simulink model "EV_Model"  (R2023b)
settings: Solver=FixedStepAuto  StartTime=0.0  StopTime=100  FixedStep=0.01  RelTol=1e-3
values from neighbouring files (symbols this model uses):
  Area = 2.3    [Data.m]
  Cd = 0.28    [Data.m]
  f = 0.01    [Data.m]
  g = 9.8    [Data.m]
  GearEff = 0.97    [Data.m]
  GearRto = 9.7    [Data.m]
  Grad = 0    [Data.m]
  MotDrvCrv_1X_rpm = [1000 2000 3000 4000 5000 6000 7000 8000 9000 10000 12000 13000 14000 15000 16000]    [Data.m]
  MotDrvCrv_1Y_Tq = [390 390 390 389 311 259 222 195 173 156 142 130 120 111 104]    [Data.m]
  MotGenCrv_1X_rpm = MotDrvCrv_1X_rpm    [Data.m]
  MotGenCrv_1Y_Tq = -1*MotDrvCrv_1Y_Tq    [Data.m]
  RotCoeff = 0.05    [Data.m]
  vhemass = 1500    [Data.m]
  WhlRollRads = 0.327    [Data.m]
libraries: simulink x2
settings Model: Creator=bingtao.hu  LastModifiedBy=bingtao.hu

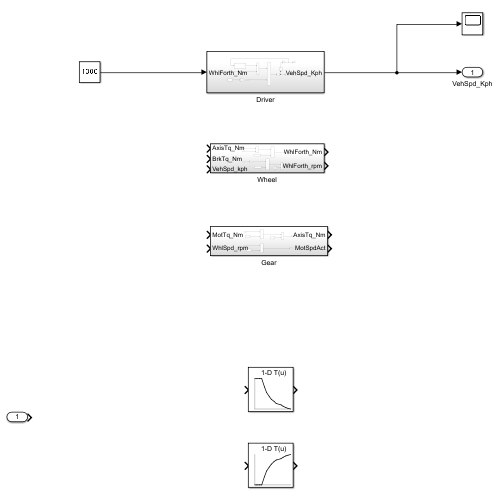
[thumbnail: Simulink's stored preview of the top-level diagram]
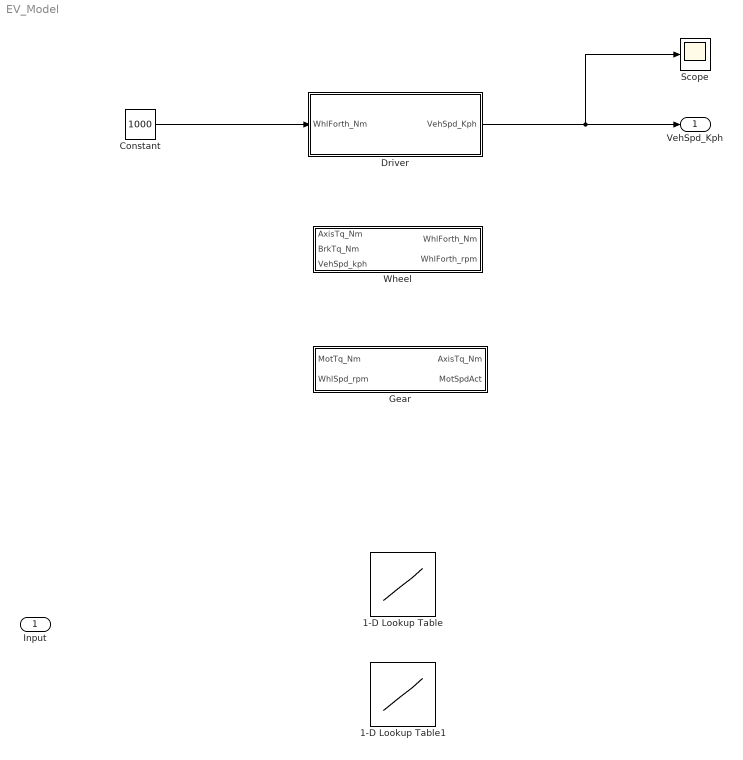
== system EV_Model ==
  Input : Inport
  1-D Lookup Table : Lookup_n-D  NumberOfTableDimensions=1  BreakpointsForDimension1=MotDrvCrv_1X_rpm  Table=MotDrvCrv_1Y_Tq  ExtrapMethod=Clip  UseLastTableValue=on  InternalRulePriority=Speed  RndMeth=Simplest
  1-D Lookup Table1 : Lookup_n-D  NumberOfTableDimensions=1  BreakpointsForDimension1=MotGenCrv_1X_rpm  Table=MotGenCrv_1Y_Tq  ExtrapMethod=Clip  UseLastTableValue=on  InternalRulePriority=Speed  RndMeth=Simplest
  Constant : Constant  Value=1000
  Driver : Subsystem
  Gear : Subsystem
  Scope : Scope
  Wheel : Subsystem
  VehSpd_Kph : Outport
  wires:
  Constant/1 -> Driver/1(WhlForth_Nm)
  Driver/1(VehSpd_Kph) -> Scope/1, VehSpd_Kph/1

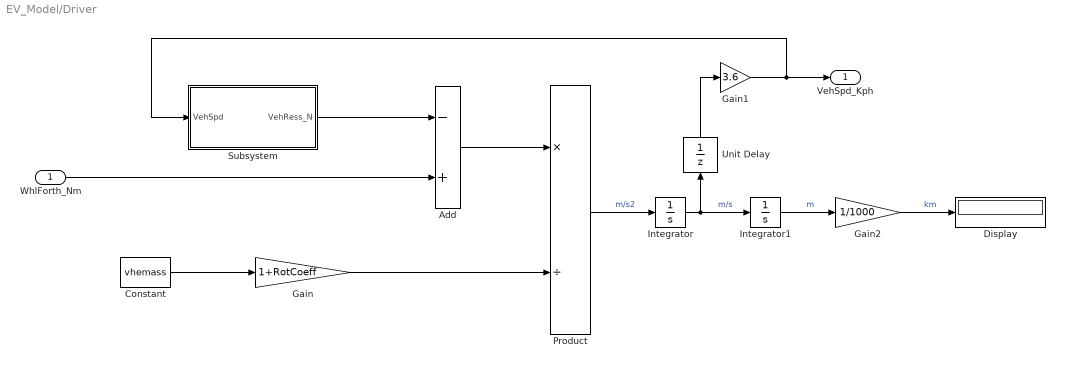
== system EV_Model/Driver ==
  WhlForth_Nm : Inport
  Add : Sum  Inputs=-+
  Constant : Constant  Value=vhemass
  Display : Display
  Gain : Gain  Gain=1+RotCoeff
  Gain1 : Gain  Gain=3.6
  Gain2 : Gain  Gain=1/1000
  Integrator : Integrator
  Integrator1 : Integrator
  Product : Product  Inputs=*/
  Subsystem : Subsystem
  Unit Delay : UnitDelay  SampleTime=-1  HasFrameUpgradeWarning=on
  VehSpd_Kph : Outport
  wires:
  WhlForth_Nm/1 -> Add/2
  Add/1 -> Product/1
  Gain1/1 -> VehSpd_Kph/1, Subsystem/1(VehSpd)
  Gain/1 -> Product/2
  Gain2/1 -> Display/1  "km"
  Subsystem/1(VehRess_N) -> Add/1
  Constant/1 -> Gain/1
  Product/1 -> Integrator/1  "m/s2"
  Integrator1/1 -> Gain2/1  "m"
  Integrator/1 -> Integrator1/1, Unit Delay/1  "m/s"
  Unit Delay/1 -> Gain1/1

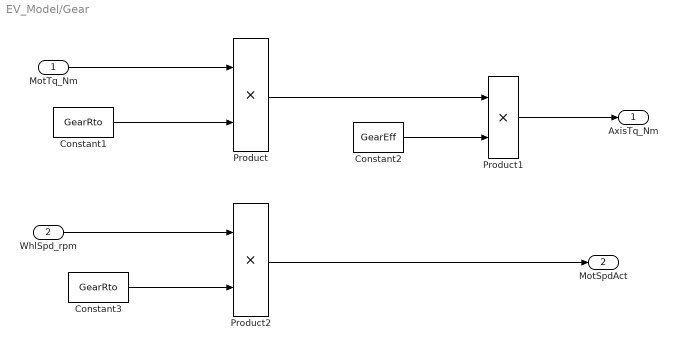
== system EV_Model/Gear ==
  MotTq_Nm : Inport
  WhlSpd_rpm : Inport  Port=2
  Constant1 : Constant  Value=GearRto
  Constant2 : Constant  Value=GearEff
  Constant3 : Constant  Value=GearRto
  Product : Product
  Product1 : Product
  Product2 : Product
  AxisTq_Nm : Outport
  MotSpdAct : Outport  Port=2
  wires:
  WhlSpd_rpm/1 -> Product2/1
  Constant1/1 -> Product/2
  Product/1 -> Product1/1
  Constant3/1 -> Product2/2
  Product1/1 -> AxisTq_Nm/1
  Constant2/1 -> Product1/2
  Product2/1 -> MotSpdAct/1
  MotTq_Nm/1 -> Product/1

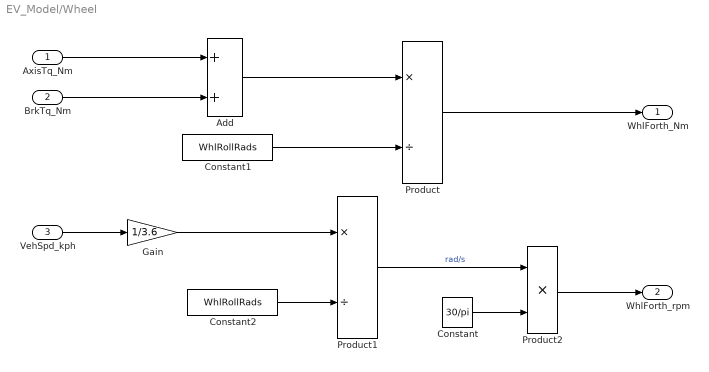
== system EV_Model/Wheel ==
  AxisTq_Nm : Inport
  BrkTq_Nm : Inport  Port=2
  VehSpd_kph : Inport  Port=3
  Add : Sum
  Constant : Constant  Value=30/pi
  Constant1 : Constant  Value=WhlRollRads
  Constant2 : Constant  Value=WhlRollRads
  Gain : Gain  Gain=1/3.6
  Product : Product  Inputs=*/
  Product1 : Product  Inputs=*/
  Product2 : Product
  WhlForth_Nm : Outport
  WhlForth_rpm : Outport  Port=2
  wires:
  BrkTq_Nm/1 -> Add/2
  AxisTq_Nm/1 -> Add/1
  Product/1 -> WhlForth_Nm/1
  Add/1 -> Product/1
  Constant1/1 -> Product/2
  VehSpd_kph/1 -> Gain/1
  Gain/1 -> Product1/1
  Constant2/1 -> Product1/2
  Product1/1 -> Product2/1  "rad/s"
  Constant/1 -> Product2/2
  Product2/1 -> WhlForth_rpm/1

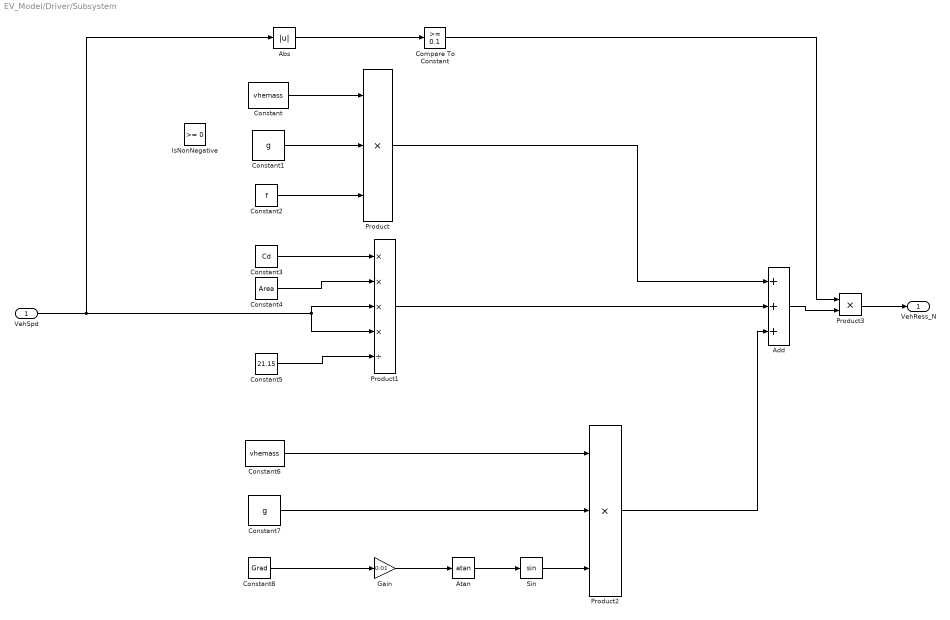
== system EV_Model/Driver/Subsystem ==
  VehSpd : Inport
  Abs : Abs  SaturateOnIntegerOverflow=off
  Add : Sum  Inputs=+++
  Atan : Trigonometry  Operator=atan
  Compare To Constant : simulink/Logic and Bit Operations/Compare To Constant  relop=>=  const=0.1  OutDataTypeStr=boolean
  Constant : Constant  Value=vhemass
  Constant1 : Constant  Value=g
  Constant2 : Constant  Value=f
  Constant3 : Constant  Value=Cd
  Constant4 : Constant  Value=Area
  Constant5 : Constant  Value=21.15
  Constant6 : Constant  Value=vhemass
  Constant7 : Constant  Value=g
  Constant8 : Constant  Value=Grad
  Gain : Gain  Gain=0.01
  IsNonNegative : simulink/Logic and Bit Operations/Compare To Zero  relop=>=  OutDataTypeStr=boolean
      settings: LibrarySourceBlock=|
      | simulink/Quick Insert/Logic and Bit
      | Operations/IsNonNegative
  Product : Product  Inputs=3
  Product1 : Product  Inputs=****/
  Product2 : Product  Inputs=3
  Product3 : Product
  Sin : Trigonometry
  VehRess_N : Outport
  wires:
  Constant5/1 -> Product1/5
  VehSpd/1 -> Abs/1, Product1/3, Product1/4
  Constant7/1 -> Product2/2
  Constant/1 -> Product/1
  Gain/1 -> Atan/1
  Constant3/1 -> Product1/1
  Constant4/1 -> Product1/2
  Atan/1 -> Sin/1
  Product2/1 -> Add/3
  Product1/1 -> Add/2
  Sin/1 -> Product2/3
  Constant6/1 -> Product2/1
  Product/1 -> Add/1
  Constant8/1 -> Gain/1
  Constant1/1 -> Product/2
  Constant2/1 -> Product/3
  Abs/1 -> Compare To Constant/1
  Compare To Constant/1 -> Product3/1
  Add/1 -> Product3/2
  Product3/1 -> VehRess_N/1
